simulink model "current_controllers"  (R2013a)
settings: Solver=ode45  StartTime=0.0  StopTime=5e-3  RelTol=1e-3
InitFcn:
  | %%%%%%  set scope time range
  | T_STOP=str2num(get_param(gcs,'StopTime'));
  | if numel(T_STOP) > 1
  |    T_STOP=T_STOP(2);
  | else
  |    T_STOP=T_STOP(1);
  | end
  | T_STOP=num2str(T_STOP);
  | 
  | %%%%%%  set scope time range in system @init_callback_fct
  | T_STOP=num2str(str2num(get_param(gcs,'StopTime')));
  | 
  | childs = allchild(0);
  | sol=strfind(upper(get(allchild(0),'Tag')),'VIEWER_PARAMETERS');
  | 
  | if iscell(sol)
  |    ind=find(~cellfun(@isempty, strfind(upper(get(allchild(0),'Tag')),'VIEWER_PARAMETERS')));
  | else
  |    ind=sol;
  | end
  | %ind=find(~cellfun(@isempty, {strfind(upper(get(allchild(0),'Tag')),'VIEWER_PARAMETERS'),[]}))
  | if ~isempty(ind)
  |    for k=1:length(childs(ind))
  |       set_param(getfield(get(childs(ind(k)),'UserData'),'block'),'TimeRange',T_STOP);
  |       get_param(getfield(get(childs(ind(k)),'UserData'),'block'),'TimeRange');
  | %    set_param(getfield(get(childs(ind),'UserData'),'block'),'TimeRange',T_STOP);
  | %    get_param(getfield(get(childs(ind),'UserData'),'block'),'TimeRange');
  |    end
  | else
  |     warning(sprintf('VIEWER_PARAMETERS object not found\nOpen the config dialog by hand for the first sim start'))
  | end
libraries: simulink x3
settings Model: Creator=mainster  LastModifiedBy=mainster

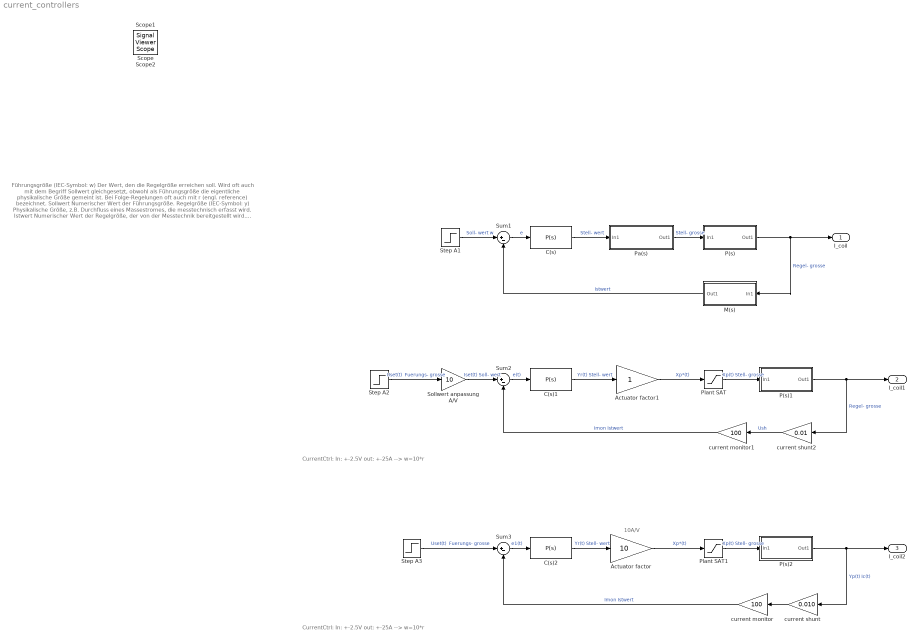
== system current_controllers ==
  note: CurrentCtrl:
      | In:		+-2.5V
      | out: 	+-25A
      | --> w=10*r
  note: Führungsgröße
      | (IEC-Symbol:  w)
      | Der Wert, den die Regelgröße erreichen soll. Wird oft auch mit dem
      | Begriff Sollwert gleichgesetzt, obwohl als Führungsgröße die
      | eigentliche physikalische Größe gemeint ist. Bei Folge-Regelungen
      | oft auch mit r (engl. reference) bezeichnet.
      |
      | Sollwert  Numerischer Wert der Führungsgröße.
      |
      | Regelgröße
      | (IEC-Symbol:  y)
      | Physikalische Größe, z.B. Durchfluss eines Massestromes, die
      | messtechnisch erfasst wird.
      |
      | Istwert
      | Numerischer Wert der Regelgröße, der von der Messtechnik
      | bereitgestellt wird.
      |
      | Regelstrecke
      | Apparativer Teil der Produktionsanlage, bei der mindestens eine
      | physikalische Größe über eine Stellgröße geregelt werden soll.
      |
      | Stellgröße
      | Physikalische Größe, mit der die Regelstrecke zum Zwecke der
      | Regelung beeinflusst wird. Dies kann z.B. elektrische Leistung oder
      | ein Dampfstrom sein.
      |
      | Stellwert
      | Numerischer Wert, der vom Regler berechnet wurde und über das
      | Stellglied die Stellgröße beeinflusst. Üblicherweise in der Einheit %
      | angegeben.
  note: CurrentCtrl:
      | In:		+-2.5V
      | out: 	+-25A
      | --> w=10*r
  note: 10A/V
  Actuator factor : Gain  Gain=10
  "Actuator factor1 " : Gain
  C(s) : simulink/Continuous/PID Controller  Controller=P  TimeDomain=Continuous-time  SampleTime=-1  IntegratorMethod=Forward Euler  FilterMethod=Forward Euler  Form=Ideal  P=3.08425264501761  I=14078.2261040339  D=0  N=100  InitialConditionSource=internal  InitialConditionForIntegrator=0  InitialConditionForFilter=0  ExternalReset=none  LimitOutput=off  UpperSaturationLimit=inf  LowerSaturationLimit=-inf  LinearizeAsGain=on  AntiWindupMode=none  Kb=1  TrackingMode=off  Kt=1  PParamMin=[]  PParamMax=[]  IParamMin=[]  IParamMax=[]  DParamMin=[]  DParamMax=[]  NParamMin=[]  NParamMax=[]  KbParamMin=[]  KbParamMax=[]  KtParamMin=[]  KtParamMax=[]  POutMin=[]  POutMax=[]  IOutMin=[]  IOutMax=[]  DOutMin=[]  DOutMax=[]  NOutMin=[]  NOutMax=[]  KbOutMin=[]  KbOutMax=[]  KtOutMin=[]  KtOutMax=[]  IntegratorOutMin=[]  IntegratorOutMax=[]  FilterOutMin=[]  FilterOutMax=[]  SumOutMin=[]  SumOutMax=[]  SumI1OutMin=[]  SumI1OutMax=[]  SumI2OutMin=[]  SumI2OutMax=[]  SumI3OutMin=[]  SumI3OutMax=[]  SumDOutMin=[]  SumDOutMax=[]  SaturationOutMin=[]  SaturationOutMax=[]  IntegratorContinuousStateAttributes=''  IntegratorStateMustResolveToSignalObject=off  IntegratorRTWStateStorageClass=Auto  FilterContinuousStateAttributes=''  FilterStateMustResolveToSignalObject=off  FilterRTWStateStorageClass=Auto  mask(PID 1dof){}
      mask Display:
      | % This is a new mask on top of the base mask.
      | % Use "View base mask" link below to see the base mask.
      | 
      | disp('Regler')
  C(s)1 : simulink/Continuous/PID Controller  Controller=P  TimeDomain=Continuous-time  SampleTime=-1  IntegratorMethod=Forward Euler  FilterMethod=Forward Euler  Form=Ideal  P=1  I=14078.2261040339  D=0  N=100  InitialConditionSource=internal  InitialConditionForIntegrator=0  InitialConditionForFilter=0  ExternalReset=none  LimitOutput=off  UpperSaturationLimit=inf  LowerSaturationLimit=-inf  LinearizeAsGain=on  AntiWindupMode=none  Kb=1  TrackingMode=off  Kt=1  PParamMin=[]  PParamMax=[]  IParamMin=[]  IParamMax=[]  DParamMin=[]  DParamMax=[]  NParamMin=[]  NParamMax=[]  KbParamMin=[]  KbParamMax=[]  KtParamMin=[]  KtParamMax=[]  POutMin=[]  POutMax=[]  IOutMin=[]  IOutMax=[]  DOutMin=[]  DOutMax=[]  NOutMin=[]  NOutMax=[]  KbOutMin=[]  KbOutMax=[]  KtOutMin=[]  KtOutMax=[]  IntegratorOutMin=[]  IntegratorOutMax=[]  FilterOutMin=[]  FilterOutMax=[]  SumOutMin=[]  SumOutMax=[]  SumI1OutMin=[]  SumI1OutMax=[]  SumI2OutMin=[]  SumI2OutMax=[]  SumI3OutMin=[]  SumI3OutMax=[]  SumDOutMin=[]  SumDOutMax=[]  SaturationOutMin=[]  SaturationOutMax=[]  IntegratorContinuousStateAttributes=''  IntegratorStateMustResolveToSignalObject=off  IntegratorRTWStateStorageClass=Auto  FilterContinuousStateAttributes=''  FilterStateMustResolveToSignalObject=off  FilterRTWStateStorageClass=Auto  mask(PID 1dof){}
      mask Display:
      | % This is a new mask on top of the base mask.
      | % Use "View base mask" link below to see the base mask.
      | 
      | disp('Regler')
  C(s)2 : simulink/Continuous/PID Controller  Controller=P  TimeDomain=Continuous-time  SampleTime=-1  IntegratorMethod=Forward Euler  FilterMethod=Forward Euler  Form=Ideal  P=1  I=14078.2261040339  D=0  N=100  InitialConditionSource=internal  InitialConditionForIntegrator=0  InitialConditionForFilter=0  ExternalReset=none  LimitOutput=off  UpperSaturationLimit=inf  LowerSaturationLimit=-inf  LinearizeAsGain=on  AntiWindupMode=none  Kb=1  TrackingMode=off  Kt=1  PParamMin=[]  PParamMax=[]  IParamMin=[]  IParamMax=[]  DParamMin=[]  DParamMax=[]  NParamMin=[]  NParamMax=[]  KbParamMin=[]  KbParamMax=[]  KtParamMin=[]  KtParamMax=[]  POutMin=[]  POutMax=[]  IOutMin=[]  IOutMax=[]  DOutMin=[]  DOutMax=[]  NOutMin=[]  NOutMax=[]  KbOutMin=[]  KbOutMax=[]  KtOutMin=[]  KtOutMax=[]  IntegratorOutMin=[]  IntegratorOutMax=[]  FilterOutMin=[]  FilterOutMax=[]  SumOutMin=[]  SumOutMax=[]  SumI1OutMin=[]  SumI1OutMax=[]  SumI2OutMin=[]  SumI2OutMax=[]  SumI3OutMin=[]  SumI3OutMax=[]  SumDOutMin=[]  SumDOutMax=[]  SaturationOutMin=[]  SaturationOutMax=[]  IntegratorContinuousStateAttributes=''  IntegratorStateMustResolveToSignalObject=off  IntegratorRTWStateStorageClass=Auto  FilterContinuousStateAttributes=''  FilterStateMustResolveToSignalObject=off  FilterRTWStateStorageClass=Auto  mask(PID 1dof){}
      mask Display:
      | % This is a new mask on top of the base mask.
      | % Use "View base mask" link below to see the base mask.
      | 
      | disp('Regler')
  M(s) : Subsystem
      mask Display: disp('Messwandler\nSensor')
  P(s) : Subsystem
      mask Display: disp('Regelstrecke\nPlant')
  P(s)1 : Subsystem
      mask Display: disp('Regelstrecke\nPlant')
  P(s)2 : Subsystem
      mask Display: disp('Regelstrecke\nPlant')
  Pa(s) : Subsystem
      mask Display: disp('Stellglied\nPlant actuator')
  Plant SAT : Saturate  UpperLimit=20  LowerLimit=-20
      settings: AttributesFormatString=I_lim=+-%<UpperLimit>A
  Plant SAT1 : Saturate  UpperLimit=20  LowerLimit=-20
      settings: AttributesFormatString=I_lim=+-%<UpperLimit>A
  Sollwert anpassung A/V : Gain  Gain=10
  Step A1 : Step  Time=1e-3  After=3  ZeroCross=off
      settings: AttributesFormatString=Ampl.: %<After>\ntime:%<Time>
  Step A2 : Step  Time=1e-3  After=0.3  ZeroCross=off
      settings: AttributesFormatString=Ampl.: %<After>V\ntime:%<Time>
  Step A3 : Step  Time=1e-3  After=0.3  ZeroCross=off
      settings: AttributesFormatString=Ampl.: %<After>V\ntime:%<Time>
  Sum1 : Sum  Inputs=|+-
  Sum2 : Sum  Inputs=|+-
  Sum3 : Sum  Inputs=|+-
  current monitor : Gain  Gain=100
  current monitor1 : Gain  Gain=100
  current shunt : Gain  Gain=0.010
  current shunt2 : Gain  Gain=0.01
  I_coil : Outport
  I_coil1 : Outport  Port=2
  I_coil2 : Outport  Port=3
  Scope : SignalViewerScope  IOType=viewer  NumInputPorts=4  RefreshTime=0.035000
      settings: ShowLegends=on  TimeRange=0.007  YMin=0~0~0~0  YMax=8~8~2.5~2.5
  Scope1 : SignalViewerScope  IOType=viewer  NumInputPorts=5  RefreshTime=0.035000
      settings: ShowLegends=on  TimeRange=0.007  YMin=0~0~0~0~0  YMax=3~3~3~1.5~1.5
  Scope2 : SignalViewerScope  IOType=viewer  NumInputPorts=5  RefreshTime=0.035000
      settings: ShowLegends=on  TimeRange=0.007  YMin=0~0~0~0~0  YMax=0.4~0.2~2~0.4~0.4  SaveName=ScopeData2
  wires:
  Sum1/1 -> C(s)/1  "e"
  C(s)/1 -> Pa(s)/1(In1)  "Stell- wert"
  Step A1/1 -> Sum1/1  "Soll- wert w"
  Pa(s)/1(Out1) -> P(s)/1(In1)  "Stell- grosse"
  P(s)/1(Out1) -> M(s)/1(In1), I_coil/1  "Regel- grosse"
  M(s)/1(Out1) -> Sum1/2  "Istwert"
  Sum2/1 -> C(s)1/1  "e(t)"
  C(s)1/1 -> "Actuator factor1 "/1  "Yr(t) Stell- wert"
  Step A2/1 -> Sollwert anpassung A/V/1  "Uset(t)  Fuerungs- grosse"
  "Actuator factor1 "/1 -> Plant SAT/1  "Xp*(t)"
  P(s)1/1(Out1) -> current shunt2/1, I_coil1/1  "Regel- grosse"
  current monitor1/1 -> Sum2/2  "Imon Istwert"
  Sollwert anpassung A/V/1 -> Sum2/1  "Iset(t) Soll- wert"
  Plant SAT/1 -> P(s)1/1(In1)  "Xp(t) Stell- grosse"
  Sum3/1 -> C(s)2/1  "e1(t)"
  C(s)2/1 -> Actuator factor/1  "Yr(t) Stell- wert"
  Step A3/1 -> Sum3/1  "Uset(t)  Fuerungs- grosse"
  Actuator factor/1 -> Plant SAT1/1  "Xp*(t)"
  P(s)2/1(Out1) -> current shunt/1, I_coil2/1  "Yp(t) Ic(t)"
  current monitor/1 -> Sum3/2  "Imon Istwert"
  Plant SAT1/1 -> P(s)2/1(In1)  "Xp(t) Stell- grosse"
  current shunt/1 -> current monitor/1
  current shunt2/1 -> current monitor1/1  "Ush"

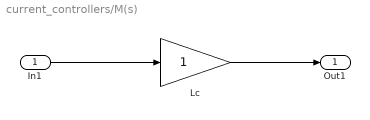
== system current_controllers/M(s) ==
  In1 : Inport
  Lc : Gain
  Out1 : Outport
  wires:
  In1/1 -> Lc/1
  Lc/1 -> Out1/1

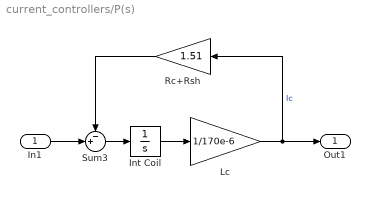
== system current_controllers/P(s) ==
  In1 : Inport
  Int Coil : Integrator
  Lc : Gain  Gain=1/170e-6
  Rc+Rsh : Gain  Gain=1.51
  Sum3 : Sum  Inputs=-+|
  Out1 : Outport
  wires:
  In1/1 -> Sum3/2
  Sum3/1 -> Int Coil/1
  Int Coil/1 -> Lc/1
  Lc/1 -> Rc+Rsh/1, Out1/1  "Ic"
  Rc+Rsh/1 -> Sum3/1

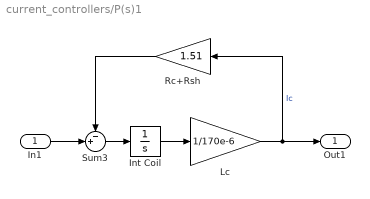
== system current_controllers/P(s)1 ==
  In1 : Inport
  Int Coil : Integrator
  Lc : Gain  Gain=1/170e-6
  Rc+Rsh : Gain  Gain=1.51
  Sum3 : Sum  Inputs=-+|
  Out1 : Outport
  wires:
  In1/1 -> Sum3/2
  Sum3/1 -> Int Coil/1
  Int Coil/1 -> Lc/1
  Lc/1 -> Rc+Rsh/1, Out1/1  "Ic"
  Rc+Rsh/1 -> Sum3/1

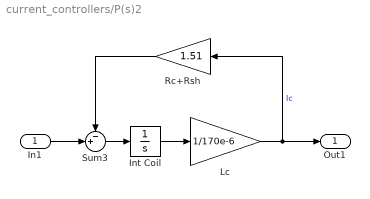
== system current_controllers/P(s)2 ==
  In1 : Inport
  Int Coil : Integrator
  Lc : Gain  Gain=1/170e-6
  Rc+Rsh : Gain  Gain=1.51
  Sum3 : Sum  Inputs=-+|
  Out1 : Outport
  wires:
  In1/1 -> Sum3/2
  Sum3/1 -> Int Coil/1
  Int Coil/1 -> Lc/1
  Lc/1 -> Rc+Rsh/1, Out1/1  "Ic"
  Rc+Rsh/1 -> Sum3/1

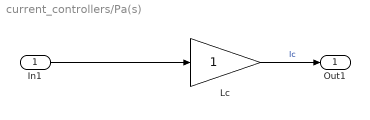
== system current_controllers/Pa(s) ==
  In1 : Inport
  Lc : Gain
  Out1 : Outport
  wires:
  In1/1 -> Lc/1
  Lc/1 -> Out1/1  "Ic"
